simulink model "Q2"  (R2024b)
settings: Solver=VariableStepAuto  StartTime=0.0  StopTime=3  RelTol=1e-3
settings Model: Creator=User  LastModifiedBy=User

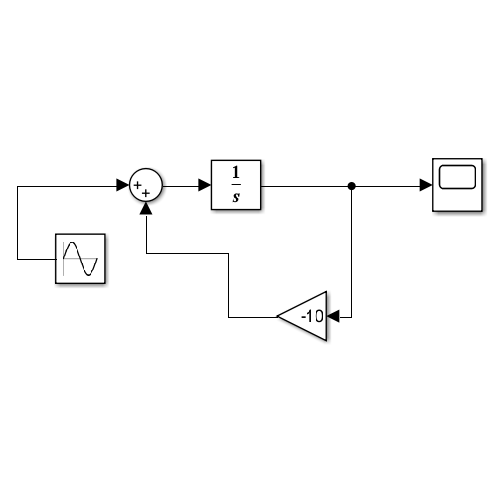
[thumbnail: Simulink's stored preview of the top-level diagram]
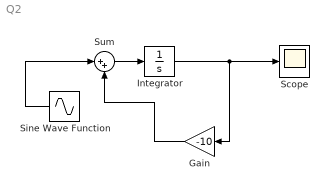
== system Q2 ==
  Gain : Gain  Gain=-10
  Integrator : Integrator  InitialCondition=1
  Scope : Scope
  Sine Wave Function : Sin  Amplitude=2  Frequency=4  SampleTime=0
  Sum : Sum  Inputs=|++
  wires:
  Integrator/1 -> Scope/1, Gain/1
  Sine Wave Function/1 -> Sum/1
  Gain/1 -> Sum/2
  Sum/1 -> Integrator/1
